simulink model "nms_model_mld"  (R2020a)
settings: Solver=VariableStepAuto  StartTime=0.0  StopTime=10  FixedStep=0.0001  MaxStep=.01  RelTol=1e-4  AbsTol=1e-6
undefined symbols (not defined in the file): animFrameRate, dt_visual, footMass, g, hatLeftHipToCenterDistWidth, hatMass, initialTargetAngle, legMass, LongDelay, LongLoopDelay, LPreStimBFSHinit, LPreStimGASinit, LPreStimGLUinit, LPreStimHABinit, LPreStimHADinit, LPreStimHAMinit, LPreStimHFLinit, LPreStimRFinit, LPreStimSOLinit, LPreStimTAinit, LPreStimVASinit, LTargetAngleInit, LTargetAngleRInit, MidDelay, params, RPreStimBFSHinit, RPreStimGASinit, RPreStimGLUinit, RPreStimHABinit, RPreStimHADinit, RPreStimHAMinit, RPreStimHFLinit, RPreStimRFinit, RPreStimSOLinit, RPreStimTAinit, RPreStimVASinit, RTargetAngleInit, RTargetAngleRInit, shankLength, shankMass, ShortDelay, termination_height, testInterpretedFnc, thetaHATref, thighLength, thighMass, totalMass, X, Y, Z
libraries: NeuroMuscularLibrary x113, nesl_utility x31, sm_lib x25, simulink x3
(part 4 of 5)

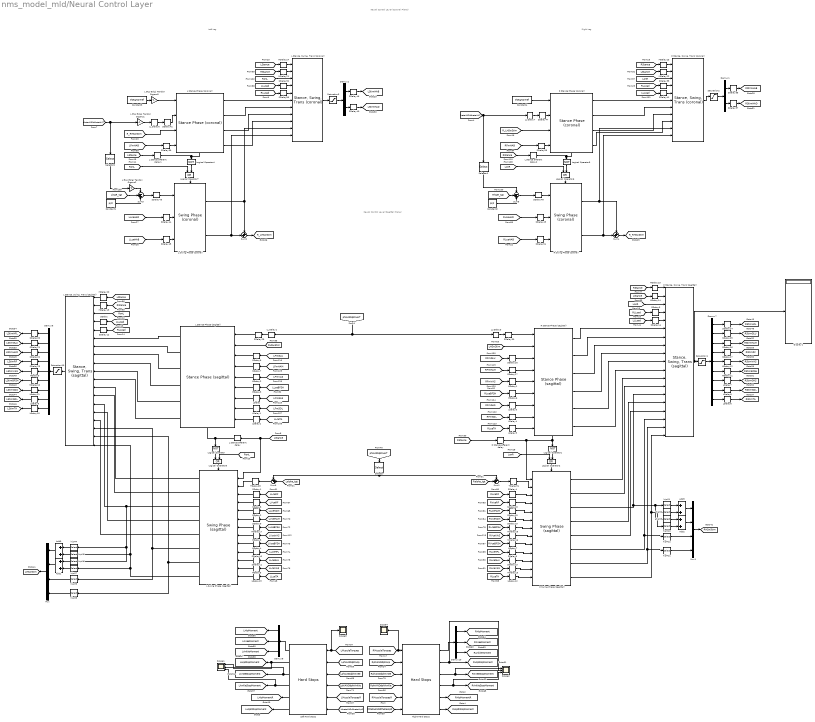
== system nms_model_mld/Neural Control Layer ==
  note: Neural Control Layer
      | (Sagittal Plane)
  note: Neural Control Layer
      | (Coronal Plane)
  note: Right Leg
  note: Left Leg
  Add{1..3,9} (4 alike) : Sum  Inputs=2
  Constant1 : Constant  Value=pi/2
  Constant2 : Constant  Value=pi/2
  Constant3 : Constant  Value=thetaHATref
  Constant4 : Constant  Value=thetaHATref
  Demux1 : Demux  Outputs=2
  Demux10 : Demux  Outputs=3
  Demux2 : Demux  Outputs=2
  Demux6 : Demux  Outputs=9
  Demux7 : Demux  Outputs=9
  Demux8 : Demux  Outputs=3
  Display1 : Display
  L GLU Golgi Tendon Organs1 : Gain  Gain=-1
  L GLU Golgi Tendon Organs2 : Gain  Gain=-1
  L GLU Golgi Tendon Organs3 : Gain  Gain=-1
  L Stance afferent delay : TransportDelay  DelayTime=MidDelay
  L Stance afferent delay1 : TransportDelay  DelayTime=MidDelay
  L Stance afferent delay2 : TransportDelay  DelayTime=MidDelay
  L Stance Phase (coronal) : NeuroMuscularLibrary/Stance Phase (coronal)  PreStimHABst=PreStimHABst  PreStimHADst=PreStimHADst  GainFHABst=GainFHABst  GainPhiHATHABst=GainPhiHATHABst  GainDphiHATHABst=GainDphiHATHABst  GainPhiHATHADst=GainPhiHATHADst  GainDphiHATHADst=GainDphiHATHADst  GainSHABcHABst=GainSHABcHABst  GainSHADcHADst=GainSHADcHADst
  L Stance Phase (sagittal) : NeuroMuscularLibrary/Stance Phase (sagittal)  PreStimHFLst=PreStimHFLst  PreStimGLUst=PreStimGLUst  PreStimHAMst=PreStimHAMst  PreStimRFst=PreStimRFst  PreStimVASst=PreStimVASst  PreStimBFSHst=PreStimBFSHst  PreStimGASst=PreStimGASst  PreStimSOLst=PreStimSOLst  PreStimTAst=PreStimTAst  GainFGLUst=GainFGLUst  GainFVASst=GainFVASst  GainFSOLst=GainFSOLst  GainFHAMst=GainFHAMst  LceOffsetBFSHVASst=LceOffsetBFSHVASst  GainLBFSHVASst=GainLBFSHVASst  LceOffsetBFSHst=LceOffsetBFSHst  GainLBFSHst=GainLBFSHst  GainFGASst=GainFGASst  phiHATref=phiHATref  GainPhiHATHFLst=GainPhiHATHFLst  GainDphiHATHFLst=GainDphiHATHFLst  GainPhiHATGLUst=GainPhiHATGLUst  GainDphiHATGLUst=GainDphiHATGLUst  GainSGLUHAMst=GainSGLUHAMst  GainSGLUcHFLst=GainSGLUcHFLst  GainSHAMcHFLst=GainSHAMcHFLst  GainSHFLcGLUst=GainSHFLcGLUst  GainSRFcGLUst=GainSRFcGLUst  LceOffsetTAst=LceOffsetTAst  GainLTAst=GainLTAst  GainFSOLTAst=GainFSOLTAst
  "L Stance, Swing, Trans (coronal)" : NeuroMuscularLibrary/Stance, Swing, Trans (coronal)  transSupst_C=transSupst_C  transsw_C=transsw_C
  "L Stance, Swing, Trans (sagittal)" : NeuroMuscularLibrary/Stance, Swing, Trans (sagittal)  transSupst=transSupst  transsw=transsw
  L Swing Phase (coronal) : NeuroMuscularLibrary/Swing Phase (coronal)  PreStimHABsw=PreStimHABsw  PreStimHADsw=PreStimHADsw  GainLHABsw=GainLHABsw  GainLHADsw=GainLHADsw
  L Swing Phase (sagittal) : NeuroMuscularLibrary/Swing Phase (sagittal)  PreStimHFLsw=PreStimHFLsw  PreStimGLUsw=PreStimGLUsw  PreStimHAMsw=PreStimHAMsw  PreStimRFsw=PreStimRFsw  PreStimVASsw=PreStimVASsw  PreStimBFSHsw=PreStimBFSHsw  PreStimGASsw=PreStimGASsw  PreStimSOLsw=PreStimSOLsw  PreStimTAsw=PreStimTAsw  GainLTAsw=GainLTAsw  LceOffsetTAsw=LceOffsetTAsw  GainLRFHFLsw=GainLRFHFLsw  GainVRFHFLsw=GainVRFHFLsw  GainLHAMGLUsw=GainLHAMGLUsw  GainVHAMGLUsw=GainVHAMGLUsw  GainVRFBFSHsw=GainVRFBFSHsw  GainVVASRFsw=GainVVASRFsw  GainVBFSHsw=GainVBFSHsw  GainLHAMsw=GainLHAMsw  GainSHAMBFSHsw=GainSHAMBFSHsw  GainSHAMGASsw=GainSHAMGASsw  SHAMthresholdsw=SHAMthresholdsw  GainLHFLsw=GainLHFLsw  GainLGLUsw=GainLGLUsw  LceOffsetVASsw=LceOffsetVASsw  GainLVASsw=GainLVASsw  legLengthClr=legLengthClr  deltaLegAngleThr=deltaLegAngleThr
  LDelay{,1,3..4} (4 alike) : TransportDelay  DelayTime=LongDelay
  LDelay10 : TransportDelay  DelayTime=LongDelay  InitialOutput=LPreStimTAinit
  LDelay11 : TransportDelay  DelayTime=LongDelay  InitialOutput=LPreStimGASinit
  LDelay{2,5,12..13} (4 alike) : TransportDelay  DelayTime=LongDelay  InitialOutput=1
  LDelay6 : TransportDelay  DelayTime=LongDelay  InitialOutput=RPreStimTAinit
  LDelay7 : TransportDelay  DelayTime=LongDelay  InitialOutput=RPreStimGASinit
  LDelay8 : TransportDelay  DelayTime=LongDelay  InitialOutput=RPreStimSOLinit
  LDelay9 : TransportDelay  DelayTime=LongDelay  InitialOutput=LPreStimSOLinit
  LL Delay{2..3,6..7} (4 alike) : TransportDelay  DelayTime=LongLoopDelay/2
  Left Hard Stops : NeuroMuscularLibrary/Hard Stops  SystemSampleTime=-1  Latency=0  AutoFrameSizeCalculation=off
  Logical Operator{,1,4..5} (4 alike) : Logic  Operator=NOT  AllPortsSameDT=off  OutDataTypeStr=boolean
  Logical Operator{2..3,6..7} (4 alike) : Logic  Operator=OR  AllPortsSameDT=off  OutDataTypeStr=boolean
  MDelay{1..2,4,7..8,13..14,16,19..24} (14 alike) : TransportDelay  DelayTime=MidDelay
  MDelay10 : TransportDelay  DelayTime=MidDelay  InitialOutput=LPreStimBFSHinit
  MDelay11 : TransportDelay  DelayTime=MidDelay  InitialOutput=RPreStimBFSHinit
  MDelay12 : TransportDelay  DelayTime=MidDelay  InitialOutput=RPreStimVASinit
  MDelay{3,5..6,15,17..18} (6 alike) : TransportDelay  DelayTime=MidDelay  InitialOutput=1
  MDelay9 : TransportDelay  DelayTime=MidDelay  InitialOutput=LPreStimVASinit
  Mux : Mux
  Mux1 : Mux
  R Stance afferent delay : TransportDelay  DelayTime=MidDelay
  R Stance Phase (coronal) : NeuroMuscularLibrary/Stance Phase (coronal)  PreStimHABst=PreStimHABst  PreStimHADst=PreStimHADst  GainFHABst=GainFHABst  GainPhiHATHABst=GainPhiHATHABst  GainDphiHATHABst=GainDphiHATHABst  GainPhiHATHADst=GainPhiHATHADst  GainDphiHATHADst=GainDphiHATHADst  GainSHABcHABst=GainSHABcHABst  GainSHADcHADst=GainSHADcHADst
  R Stance Phase (sagittal) : NeuroMuscularLibrary/Stance Phase (sagittal)  PreStimHFLst=PreStimHFLst  PreStimGLUst=PreStimGLUst  PreStimHAMst=PreStimHAMst  PreStimRFst=PreStimRFst  PreStimVASst=PreStimVASst  PreStimBFSHst=PreStimBFSHst  PreStimGASst=PreStimGASst  PreStimSOLst=PreStimSOLst  PreStimTAst=PreStimTAst  GainFGLUst=GainFGLUst  GainFVASst=GainFVASst  GainFSOLst=GainFSOLst  GainFHAMst=GainFHAMst  LceOffsetBFSHVASst=LceOffsetBFSHVASst  GainLBFSHVASst=GainLBFSHVASst  LceOffsetBFSHst=LceOffsetBFSHst  GainLBFSHst=GainLBFSHst  GainFGASst=GainFGASst  phiHATref=phiHATref  GainPhiHATHFLst=GainPhiHATHFLst  GainDphiHATHFLst=GainDphiHATHFLst  GainPhiHATGLUst=GainPhiHATGLUst  GainDphiHATGLUst=GainDphiHATGLUst  GainSGLUHAMst=GainSGLUHAMst  GainSGLUcHFLst=GainSGLUcHFLst  GainSHAMcHFLst=GainSHAMcHFLst  GainSHFLcGLUst=GainSHFLcGLUst  GainSRFcGLUst=GainSRFcGLUst  LceOffsetTAst=LceOffsetTAst  GainLTAst=GainLTAst  GainFSOLTAst=GainFSOLTAst
  "R Stance, Swing, Trans (coronal)" : NeuroMuscularLibrary/Stance, Swing, Trans (coronal)  transSupst_C=transSupst_C  transsw_C=transsw_C
  "R Stance, Swing, Trans (sagittal)" : NeuroMuscularLibrary/Stance, Swing, Trans (sagittal)  transSupst=transSupst  transsw=transsw
  R Swing Phase (coronal) : NeuroMuscularLibrary/Swing Phase (coronal)  PreStimHABsw=PreStimHABsw  PreStimHADsw=PreStimHADsw  GainLHABsw=GainLHABsw  GainLHADsw=GainLHADsw
  R Swing Phase (sagittal) : NeuroMuscularLibrary/Swing Phase (sagittal)  PreStimHFLsw=PreStimHFLsw  PreStimGLUsw=PreStimGLUsw  PreStimHAMsw=PreStimHAMsw  PreStimRFsw=PreStimRFsw  PreStimVASsw=PreStimVASsw  PreStimBFSHsw=PreStimBFSHsw  PreStimGASsw=PreStimGASsw  PreStimSOLsw=PreStimSOLsw  PreStimTAsw=PreStimTAsw  GainLTAsw=GainLTAsw  LceOffsetTAsw=LceOffsetTAsw  GainLRFHFLsw=GainLRFHFLsw  GainVRFHFLsw=GainVRFHFLsw  GainLHAMGLUsw=GainLHAMGLUsw  GainVHAMGLUsw=GainVHAMGLUsw  GainVRFBFSHsw=GainVRFBFSHsw  GainVVASRFsw=GainVVASRFsw  GainVBFSHsw=GainVBFSHsw  GainLHAMsw=GainLHAMsw  GainSHAMBFSHsw=GainSHAMBFSHsw  GainSHAMGASsw=GainSHAMGASsw  SHAMthresholdsw=SHAMthresholdsw  GainLHFLsw=GainLHFLsw  GainLGLUsw=GainLGLUsw  LceOffsetVASsw=LceOffsetVASsw  GainLVASsw=GainLVASsw  legLengthClr=legLengthClr  deltaLegAngleThr=deltaLegAngleThr
  Right Hard Stops : NeuroMuscularLibrary/Hard Stops  SystemSampleTime=-1  Latency=0  AutoFrameSizeCalculation=off
  SDelay{,3,6..9,12,14,16..19,29..30,32..33,36,38..39,41..42,47} (22 alike) : TransportDelay  DelayTime=ShortDelay
  SDelay{1..2,4..5,10..11,13,15,34,44..45,49} (12 alike) : TransportDelay  DelayTime=ShortDelay  InitialOutput=1
  SDelay20 : TransportDelay  DelayTime=ShortDelay  InitialOutput=LPreStimHFLinit
  SDelay21 : TransportDelay  DelayTime=ShortDelay  InitialOutput=LPreStimGLUinit
  SDelay22 : TransportDelay  DelayTime=ShortDelay  InitialOutput=LPreStimHAMinit
  SDelay23 : TransportDelay  DelayTime=ShortDelay  InitialOutput=LPreStimRFinit
  SDelay24 : TransportDelay  DelayTime=ShortDelay  InitialOutput=RPreStimHFLinit
  SDelay25 : TransportDelay  DelayTime=ShortDelay  InitialOutput=RPreStimGLUinit
  SDelay26 : TransportDelay  DelayTime=ShortDelay  InitialOutput=RPreStimHAMinit
  SDelay27 : TransportDelay  DelayTime=ShortDelay  InitialOutput=RPreStimRFinit
  SDelay35 : TransportDelay  DelayTime=ShortDelay  InitialOutput=RPreStimHABinit
  SDelay37 : TransportDelay  DelayTime=ShortDelay  InitialOutput=RPreStimHADinit
  SDelay40 : TransportDelay  DelayTime=ShortDelay  InitialOutput=LPreStimHADinit
  SDelay43 : TransportDelay  DelayTime=(ShortDelay + LongLoopDelay/2)  InitialOutput=LTargetAngleRInit
  SDelay46 : TransportDelay  DelayTime=ShortDelay  InitialOutput=LPreStimHABinit
  SDelay48 : TransportDelay  DelayTime=(ShortDelay + LongLoopDelay/2)  InitialOutput=RTargetAngleRInit
  Saturation{1..3,10} (4 alike) : Saturate  UpperLimit=1  LowerLimit=0.01  ZeroCross=off
  Scope1 : Scope  NumInputPorts=3
  Scope2 : Scope  NumInputPorts=3
  Scope3 : Scope
  Scope4 : Scope
  Selector : Selector  InputPortWidth=2  IndexOptions=Index vector (dialog)  Indices=[1]  OutputSizes=1
  Selector1 : Selector  InputPortWidth=2  IndexOptions=Index vector (dialog)  Indices=[1]  OutputSizes=1
  Selector2 : Selector  InputPortWidth=2  IndexOptions=Index vector (dialog)  Indices=[1]  OutputSizes=1
  Sum1 : Sum  Inputs=-+|
  Sum2 : Sum  Inputs=++|
  Sum3 : Sum  Inputs=--+
  Sum4 : Sum  Inputs=++|
  Sum5 : Sum  Inputs=--+
  Sum6 : Sum  Inputs=-+|
  TDelay28 : TransportDelay  DelayTime=(ShortDelay + LongLoopDelay/2)  InitialOutput=LTargetAngleInit
  TDelay31 : TransportDelay  DelayTime=(ShortDelay + LongLoopDelay/2)  InitialOutput=RTargetAngleInit
  hipM{1,4,9,12} (4 alike) : Selector  InputPortWidth=2  IndexOptions=Index vector (dialog)  Indices=1  OutputSizes=1
  hipM10 : Selector  InputPortWidth=3  IndexOptions=Index vector (dialog)  Indices=2  OutputSizes=1
  hipM{2,5,8,11} (4 alike) : Selector  InputPortWidth=3  IndexOptions=Index vector (dialog)  Indices=1  OutputSizes=1
  hipM3 : Selector  InputPortWidth=2  IndexOptions=Index vector (dialog)  Indices=2  OutputSizes=1
  hipM6 : Selector  InputPortWidth=2  IndexOptions=Index vector (dialog)  Indices=2  OutputSizes=1
  hipM7 : Selector  InputPortWidth=3  IndexOptions=Index vector (dialog)  Indices=2  OutputSizes=1
  tag scope: LAnkleMoment=global, LAnkleStopMoment=global, LHSwStim=global, LHipMoment=global, LHipMomentR=global, LHipRStopMoment=global, LHipStopMoment=global, LKneeMoment=global, LKneeStopMoment=global, LStimBFSH=global, LStimGAS=global, LStimGLU=global, LStimHAB=global, LStimHAD=global, LStimHAM=global, LStimHFL=global, LStimRF=global, LStimSOL=global, LStimTA=global, LStimVAS=global, RAnkleMoment=global, RAnkleStopMoment=global, RHSwStim=global, RHipMoment=global, RHipMomentR=global, RHipRStopMoment=global, RHipStopMoment=global, RKneeMoment=global, RKneeStopMoment=global, RStimBFSH=global, RStimGAS=global, RStimGLU=global, RStimHAB=global, RStimHAD=global, RStimHAM=global, RStimHFL=global, RStimRF=global, RStimSOL=global, RStimTA=global, RStimVAS=global, R_LHSwStim=global, R_RHSwStim=global
  wires:
  LDelay11/1 -> [LStimGAS]
  [RLceVAS] -> MDelay15/1
  LDelay10/1 -> [LStimTA]
  L Swing Phase (sagittal)/7 -> "L Stance, Swing, Trans (sagittal)"/18, hipM8/1
  Mux/1 -> [LHSwStim]
  hipM2/1 -> Add3/2
  SDelay11/1 -> L Swing Phase (sagittal)/11
  MDelay16/1 -> R Swing Phase (sagittal)/8
  SDelay24/1 -> [RStimHFL]
  [RLceRF] -> SDelay4/1
  MDelay19/1 -> "L Stance, Swing, Trans (sagittal)"/2
  SDelay10/1 -> L Swing Phase (sagittal)/10
  hipM10/1 -> Add2/2
  R Stance Phase (sagittal)/5 -> "R Stance, Swing, Trans (sagittal)"/10
  hipM4/1 -> Add9/1
  SDelay2/1 -> L Swing Phase (sagittal)/5
  [RLceBFSH] -> MDelay6/1
  [RLceGLU] -> SDelay13/1
  L Swing Phase (sagittal)/1 -> "L Stance, Swing, Trans (sagittal)"/12
  LDelay/1 -> L Stance Phase (sagittal)/7
  L Stance Phase (sagittal)/1 -> "L Stance, Swing, Trans (sagittal)"/6
  SDelay9/1 -> L Swing Phase (sagittal)/6
  L Swing Phase (sagittal)/3 -> "L Stance, Swing, Trans (sagittal)"/14, hipM6/1, hipM4/1
  R Swing Phase (sagittal)/7 -> "R Stance, Swing, Trans (sagittal)"/18, hipM11/1
  R Swing Phase (sagittal)/4 -> "R Stance, Swing, Trans (sagittal)"/15
  Add2/1 -> Mux1/2
  L Swing Phase (sagittal)/5 -> "L Stance, Swing, Trans (sagittal)"/16
  SDelay14/1 -> "R Stance, Swing, Trans (sagittal)"/5
  Demux6/2 -> SDelay21/1
  R Stance Phase (sagittal)/2 -> "R Stance, Swing, Trans (sagittal)"/7
  SDelay12/1 -> "L Stance, Swing, Trans (sagittal)"/5
  MDelay2/1 -> L Stance Phase (sagittal)/5
  Sum1/1 -> TDelay31/1
  Demux7/8 -> LDelay8/1
  hipM6/1 -> Add1/1
  R Stance Phase (sagittal)/3 -> "R Stance, Swing, Trans (sagittal)"/8
  LDelay9/1 -> [LStimSOL]
  Demux6/1 -> SDelay20/1
  L Stance Phase (sagittal)/6 -> "L Stance, Swing, Trans (sagittal)"/11
  SDelay4/1 -> R Swing Phase (sagittal)/3
  [RVceVAS] -> MDelay16/1
  hipM11/1 -> Mux1/4
  MDelay8/1 -> L Swing Phase (sagittal)/8
  Add3/1 -> Mux1/1
  R Swing Phase (sagittal)/6 -> "R Stance, Swing, Trans (sagittal)"/17, hipM12/1
  "R Stance, Swing, Trans (sagittal)"/1 -> Display1/1, Saturation1/1
  [RVceBFSH] -> MDelay7/1
  Add1/1 -> Mux/2
  hipM9/1 -> Mux/3
  L Stance Phase (sagittal)/3 -> "L Stance, Swing, Trans (sagittal)"/8
  LDelay8/1 -> [RStimSOL]
  Logical Operator2/1 -> R Swing Phase (sagittal)/Enable
  hipM5/1 -> Add9/2
  MDelay20/1 -> "L Stance, Swing, Trans (sagittal)"/1
  L Swing Phase (sagittal)/2 -> "L Stance, Swing, Trans (sagittal)"/13
  hipM8/1 -> Mux/4
  L Swing Phase (sagittal)/4 -> "L Stance, Swing, Trans (sagittal)"/15
  L Swing Phase (sagittal)/8 -> "L Stance, Swing, Trans (sagittal)"/19, hipM5/1, hipM7/1
  [LStance] -> MDelay20/1
  R Stance Phase (sagittal)/4 -> "R Stance, Swing, Trans (sagittal)"/9
  LL Delay3/1 -> SDelay30/1
  SDelay30/1 -> R Stance Phase (sagittal)/1
  SDelay22/1 -> [LStimHAM]
  SDelay29/1 -> L Stance Phase (sagittal)/1
  TDelay28/1 -> L Swing Phase (sagittal)/2
  hipM1/1 -> Add3/1
  R Stance Phase (sagittal)/6 -> "R Stance, Swing, Trans (sagittal)"/11
  R Swing Phase (sagittal)/8 -> "R Stance, Swing, Trans (sagittal)"/19, hipM2/1, hipM10/1
  Sum6/1 -> TDelay28/1
  Demux7/1 -> SDelay24/1
  [LLceGLU] -> SDelay11/1
  [RLceHFL] -> SDelay5/1
  L Stance Phase (sagittal)/2 -> "L Stance, Swing, Trans (sagittal)"/7
  R Stance Phase (sagittal)/1 -> "R Stance, Swing, Trans (sagittal)"/6
  [LLceVAS] -> MDelay5/1
  [LHSwStim] -> R Stance Phase (sagittal)/2
  SDelay/1 -> "L Stance, Swing, Trans (sagittal)"/4
  SDelay27/1 -> [RStimRF]
  MDelay11/1 -> [RStimBFSH]
  [RFmSOL] -> LDelay4/1
  MDelay10/1 -> [LStimBFSH]
  Add9/1 -> Mux/1
  [LLceHFL] -> SDelay10/1
  SDelay26/1 -> [RStimHAM]
  SDelay21/1 -> [LStimGLU]
  Demux7/6 -> MDelay11/1
  Demux7/5 -> MDelay12/1
  [LLLoad] -> SDelay14/1
  Saturation1/1 -> Demux7/1
  SDelay5/1 -> R Swing Phase (sagittal)/10
  [LFmSOL] -> LDelay1/1
  hipM12/1 -> Mux1/3
  [LonR] -> "R Stance, Swing, Trans (sagittal)"/3
  MDelay15/1 -> R Swing Phase (sagittal)/12
  [LLLoad] -> SDelay/1
  SDelay25/1 -> [RStimGLU]
  Demux7/3 -> SDelay26/1
  L Stance Phase (sagittal)/4 -> "L Stance, Swing, Trans (sagittal)"/9
  Demux7/4 -> SDelay27/1
  hipM3/1 -> Add2/1
  R Swing Phase (sagittal)/2 -> "R Stance, Swing, Trans (sagittal)"/13
  R Swing Phase (sagittal)/1 -> "R Stance, Swing, Trans (sagittal)"/12
  L Stance Phase (sagittal)/5 -> "L Stance, Swing, Trans (sagittal)"/10
  MDelay9/1 -> [LStimVAS]
  MDelay7/1 -> R Swing Phase (sagittal)/9
  SDelay3/1 -> "R Stance, Swing, Trans (sagittal)"/4
  Demux7/9 -> LDelay6/1
  TDelay31/1 -> R Swing Phase (sagittal)/2
  SDelay19/1 -> R Swing Phase (sagittal)/6
  [RVceHAM] -> SDelay19/1
  SDelay18/1 -> R Swing Phase (sagittal)/4
  SDelay15/1 -> R Swing Phase (sagittal)/5
  [RLceHAM] -> SDelay15/1
  [RLceTA] -> LDelay5/1
  LDelay7/1 -> [RStimGAS]
  LDelay3/1 -> R Stance Phase (sagittal)/7
  [RFmGAS] -> LDelay3/1
  [LLceBFSH] -> MDelay3/1
  [RFmVAS] -> MDelay1/1
  [RLLoad] -> SDelay3/1
  SDelay17/1 -> R Stance Phase (sagittal)/4
  Demux6/7 -> LDelay11/1
  [RStance] -> MDelay19/1
  Saturation10/1 -> Demux6/1
  MDelay4/1 -> L Swing Phase (sagittal)/9
  L Swing Phase (sagittal)/6 -> "L Stance, Swing, Trans (sagittal)"/17, hipM9/1
  Demux6/6 -> MDelay10/1
  Demux6/3 -> SDelay22/1
  LDelay6/1 -> [RStimTA]
  [LVceBFSH] -> MDelay4/1
  SDelay8/1 -> L Swing Phase (sagittal)/4
  Demux6/9 -> LDelay10/1
  [RVceRF] -> SDelay18/1
  Demux6/8 -> LDelay9/1
  Demux6/5 -> MDelay9/1
  MDelay5/1 -> L Swing Phase (sagittal)/12
  SDelay16/1 -> R Stance Phase (sagittal)/3
  SDelay23/1 -> [LStimRF]
  [RLLoad] -> SDelay12/1
  R Swing Phase (sagittal)/3 -> "R Stance, Swing, Trans (sagittal)"/14, hipM3/1, hipM1/1
  [LVceRF] -> SDelay8/1
  SDelay13/1 -> R Swing Phase (sagittal)/11
  Mux1/1 -> [RHSwStim]
  LDelay4/1 -> R Stance Phase (sagittal)/8
  MDelay1/1 -> R Stance Phase (sagittal)/5
  L Stance afferent delay/1 -> L Stance Phase (sagittal)/Enable, Logical Operator/1
  Logical Operator3/1 -> L Swing Phase (sagittal)/Enable
  SDelay20/1 -> [LStimHFL]
  [LLceRF] -> SDelay1/1
  [LVceHAM] -> SDelay9/1
  LDelay2/1 -> L Stance Phase (sagittal)/9
  [LLceTA] -> LDelay2/1
  Demux7/2 -> SDelay25/1
  SDelay1/1 -> L Swing Phase (sagittal)/3
  [RFmHAM] -> SDelay17/1
  Logical Operator/1 -> Logical Operator3/2
  [LLceHAM] -> SDelay2/1
  Demux6/4 -> SDelay23/1
  LDelay1/1 -> L Stance Phase (sagittal)/8
  [LFmGAS] -> LDelay/1
  [RFmGLU] -> SDelay16/1
  MDelay3/1 -> L Stance Phase (sagittal)/6
  SDelay6/1 -> L Stance Phase (sagittal)/3
  [LVceVAS] -> MDelay8/1
  [LFmVAS] -> MDelay2/1
  LL Delay2/1 -> SDelay29/1
  Demux7/7 -> LDelay7/1
  R Swing Phase (sagittal)/5 -> "R Stance, Swing, Trans (sagittal)"/16
  [LFmGLU] -> SDelay6/1
  SDelay7/1 -> L Stance Phase (sagittal)/4
  MDelay6/1 -> R Stance Phase (sagittal)/6
  MDelay12/1 -> [RStimVAS]
  [LFmHAM] -> SDelay7/1
  [RHSwStim] -> L Stance Phase (sagittal)/2
  hipM7/1 -> Add1/2
  Logical Operator1/1 -> Logical Operator2/2
  [RLceTA] -> LDelay12/1
  LDelay12/1 -> R Swing Phase (sagittal)/13
  [LLceTA] -> LDelay13/1
  MDelay17/1 -> L Swing Phase (sagittal)/7
  [LLceBFSH] -> MDelay17/1
  LDelay13/1 -> L Swing Phase (sagittal)/13
  MDelay18/1 -> R Swing Phase (sagittal)/7
  [RLceBFSH] -> MDelay18/1
  LDelay5/1 -> R Stance Phase (sagittal)/9
  R Stance afferent delay/1 -> R Swing Phase (sagittal)/1, R Stance Phase (sagittal)/Enable, Logical Operator1/1
  [RonL] -> "L Stance, Swing, Trans (sagittal)"/3
  [LonR] -> Logical Operator2/1
  [RonL] -> Logical Operator3/1
  [RStance] -> MDelay13/1
  MDelay13/1 -> "R Stance, Swing, Trans (sagittal)"/1
  [LStance] -> MDelay14/1
  MDelay14/1 -> "R Stance, Swing, Trans (sagittal)"/2
  [Ralpha_tgt] -> Sum1/2
  Selector/1 -> Sum6/1, Sum1/1
  [Lalpha_tgt] -> Sum6/2
  [phiANDdphiHAT] -> LL Delay2/1, LL Delay3/1
  [RFmHAB] -> SDelay38/1
  SDelay35/1 -> [RStimHAB]
  [LFmHAB] -> SDelay39/1
  SDelay37/1 -> [RStimHAD]
  [LLceHAD] -> SDelay44/1
  SDelay39/1 -> L Stance Phase (coronal)/4
  L Stance Phase (coronal)/2 -> "L Stance, Swing, Trans (coronal)"/7
  MDelay21/1 -> "L Stance, Swing, Trans (coronal)"/2
  L Swing Phase (coronal)/2 -> "L Stance, Swing, Trans (coronal)"/11, Sum2/2
  [LhipR_tgt] -> Sum3/2
  L GLU Golgi Tendon Organs2/1 -> Sum3/1
  Logical Operator5/1 -> Logical Operator6/2
  [RLceHAD] -> SDelay49/1
  Selector2/1 -> L GLU Golgi Tendon Organs2/1
  Logical Operator4/1 -> Logical Operator7/2
  [LLceHAB] -> SDelay45/1
  Constant4/1 -> R Stance Phase (coronal)/1
  [RonL] -> Logical Operator7/1
  Logical Operator6/1 -> R Swing Phase (coronal)/Enable
  L Swing Phase (coronal)/1 -> "L Stance, Swing, Trans (coronal)"/10, Sum2/1
  L Stance Phase (coronal)/1 -> "L Stance, Swing, Trans (coronal)"/6
  SDelay32/1 -> "L Stance, Swing, Trans (coronal)"/4
  L GLU Golgi Tendon Organs1/1 -> LL Delay6/1
  Sum3/1 -> SDelay43/1
  "L Stance, Swing, Trans (coronal)"/1 -> Saturation3/1
  SDelay43/1 -> L Swing Phase (coronal)/1
  SDelay40/1 -> [LStimHAD]
  MDelay24/1 -> "L Stance, Swing, Trans (coronal)"/1
  Selector1/1 -> Sum5/1
  L Stance afferent delay1/1 -> L Stance Phase (coronal)/Enable, Logical Operator4/1
  SDelay46/1 -> [LStimHAB]
  SDelay45/1 -> L Swing Phase (coronal)/3
  SDelay44/1 -> L Swing Phase (coronal)/2
  [RStance] -> MDelay23/1
  MDelay23/1 -> "R Stance, Swing, Trans (coronal)"/1
  SDelay49/1 -> R Swing Phase (coronal)/2
  [R_LHSwStim] -> R Stance Phase (coronal)/3
  Logical Operator7/1 -> L Swing Phase (coronal)/Enable
  Sum2/1 -> [R_LHSwStim]
  [LStance] -> L Stance afferent delay1/1
  L Stance Phase (coronal)/4 -> "L Stance, Swing, Trans (coronal)"/9
  Demux1/2 -> SDelay37/1
  SDelay42/1 -> L Stance Phase (coronal)/2
  [RonL] -> "L Stance, Swing, Trans (coronal)"/3
  L Stance afferent delay2/1 -> R Stance Phase (coronal)/Enable, Logical Operator5/1
  L Stance Phase (coronal)/3 -> "L Stance, Swing, Trans (coronal)"/8
  SDelay36/1 -> "L Stance, Swing, Trans (coronal)"/5
  Demux2/1 -> SDelay46/1
  [LLLoad] -> SDelay32/1
  [RStance] -> MDelay21/1
  [RLLoad] -> SDelay33/1
  [RStance] -> L Stance afferent delay2/1
  [LStance] -> MDelay24/1
  [LLLoad] -> SDelay41/1
  [LonR] -> Logical Operator6/1
  [RLLoad] -> SDelay36/1
  [R_RHSwStim] -> L Stance Phase (coronal)/3
  L GLU Golgi Tendon Organs3/1 -> L Stance Phase (coronal)/1
  SDelay41/1 -> "R Stance, Swing, Trans (coronal)"/5
  "R Stance, Swing, Trans (coronal)"/1 -> Saturation2/1
  SDelay47/1 -> R Stance Phase (coronal)/2
  Constant2/1 -> Sum5/3
  R Stance Phase (coronal)/2 -> "R Stance, Swing, Trans (coronal)"/7
  SDelay38/1 -> R Stance Phase (coronal)/4
  Saturation2/1 -> Demux1/1
  [LStance] -> MDelay22/1
  SDelay34/1 -> R Swing Phase (coronal)/3
  MDelay22/1 -> "R Stance, Swing, Trans (coronal)"/2
  Constant1/1 -> Sum3/3
  [LonR] -> "R Stance, Swing, Trans (coronal)"/3
  SDelay48/1 -> R Swing Phase (coronal)/1
  [RLceHAB] -> SDelay34/1
  R Stance Phase (coronal)/1 -> "R Stance, Swing, Trans (coronal)"/6
  Saturation3/1 -> Demux2/1
  R Swing Phase (coronal)/1 -> "R Stance, Swing, Trans (coronal)"/10, Sum4/1
  LL Delay7/1 -> SDelay47/1
  R Stance Phase (coronal)/3 -> "R Stance, Swing, Trans (coronal)"/8
  LL Delay6/1 -> SDelay42/1
  R Stance Phase (coronal)/4 -> "R Stance, Swing, Trans (coronal)"/9
  Demux1/1 -> SDelay35/1
  Demux2/2 -> SDelay40/1
  R Swing Phase (coronal)/2 -> "R Stance, Swing, Trans (coronal)"/11, Sum4/2
  SDelay33/1 -> "R Stance, Swing, Trans (coronal)"/4
  Sum4/1 -> [R_RHSwStim]
  [RhipR_tgt] -> Sum5/2
  Constant3/1 -> L GLU Golgi Tendon Organs3/1
  "L Stance, Swing, Trans (sagittal)"/1 -> Saturation10/1
  [RphiANDdphiHip] -> Right Hard Stops/2
  Demux10/2 -> [RKneeMoment]
  [RphiANDdphiAnkle] -> Right Hard Stops/4
  [LMuscleTorques] -> Scope3/1, Left Hard Stops/1
  [LphiANDdphiAnkle] -> Left Hard Stops/4
  [LphiANDdphiKnee] -> Left Hard Stops/3
  [RMuscleTorques] -> Scope4/1, Right Hard Stops/1
  [LphiANDdphiHip] -> Left Hard Stops/2
  Right Hard Stops/1 -> Demux10/1
  Left Hard Stops/1 -> Demux8/1
  Right Hard Stops/3 -> Scope2/2, [RKneeStopMoment]
  Demux10/1 -> [RHipMoment]
  Demux10/3 -> [RAnkleMoment]
  Left Hard Stops/4 -> Scope1/3, [LAnkleStopMoment]
  Right Hard Stops/2 -> Scope2/1, [RHipStopMoment]
  Left Hard Stops/3 -> [LKneeStopMoment], Scope1/2
  Right Hard Stops/4 -> [RAnkleStopMoment], Scope2/3
  Demux8/2 -> [LKneeMoment]
  Left Hard Stops/2 -> Scope1/1, [LHipStopMoment]
  Demux8/1 -> [LHipMoment]
  Demux8/3 -> [LAnkleMoment]
  [RphiANDdphiKnee] -> Right Hard Stops/3
  [LMuscleTorquesR] -> Left Hard Stops/5
  [RMuscleTorquesR] -> Right Hard Stops/5
  Left Hard Stops/5 -> [LHipMomentR]
  Right Hard Stops/5 -> [RHipMomentR]
  [LthetaANDdthetaHipR] -> Left Hard Stops/6
  [RthetaANDdthetaHipR] -> Right Hard Stops/6
  Left Hard Stops/6 -> [LHipRStopMoment]
  Right Hard Stops/6 -> [RHipRStopMoment]
  [phiANDdphiHAT] -> Selector/1
  [thetaANDdthetaHAT] -> LL Delay7/1, Selector1/1
  [thetaANDdthetaHAT] -> L GLU Golgi Tendon Organs1/1, Selector2/1
  [LStance] -> L Swing Phase (sagittal)/1, L Stance afferent delay/1
  [RStance] -> R Stance afferent delay/1
  Sum5/1 -> SDelay48/1

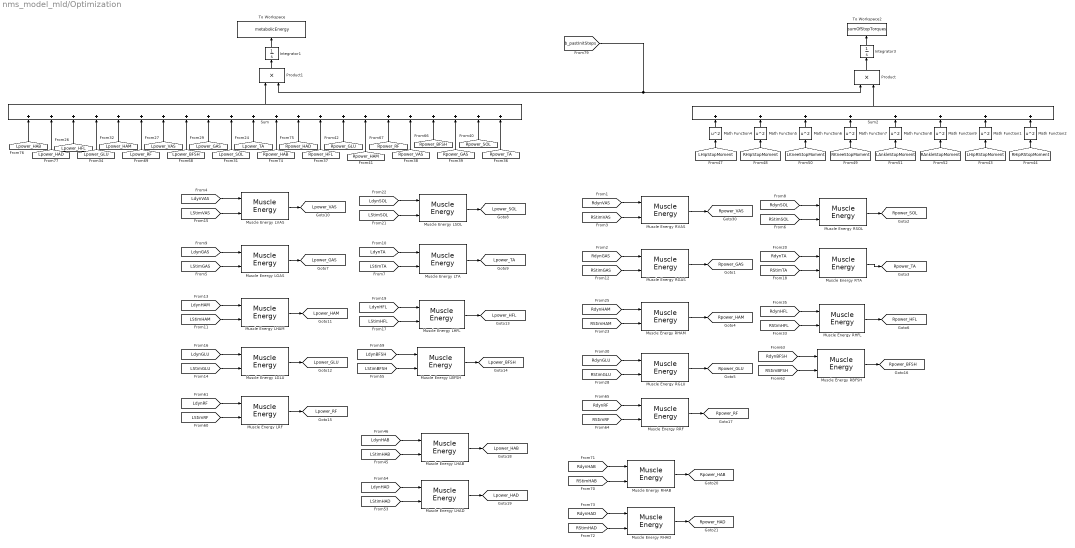
== system nms_model_mld/Optimization ==
  Integrator1 : Integrator
  Integrator3 : Integrator
  Math Function{1..2,4..9} (8 alike) : Math  Operator=square  SignedPower=on  SaturateOnIntegerOverflow=on
  Muscle Energy LBFSH : NeuroMuscularLibrary/Muscle Energy  lopt=loptBFSH  FT=FT_BFSH  Fmax=FmaxBFSH  vmax=vmaxBFSH
  Muscle Energy LGAS : NeuroMuscularLibrary/Muscle Energy  lopt=loptGAS  FT=FT_GAS  Fmax=FmaxGAS  vmax=vmaxGAS
  Muscle Energy LGLU : NeuroMuscularLibrary/Muscle Energy  lopt=loptGLU  FT=FT_GLU  Fmax=FmaxGLU  vmax=vmaxGLU
  Muscle Energy LHAB : NeuroMuscularLibrary/Muscle Energy  lopt=loptHAB  FT=FT_HAB  Fmax=FmaxHAB  vmax=vmaxHAB
  Muscle Energy LHAD : NeuroMuscularLibrary/Muscle Energy  lopt=loptHAD  FT=FT_HAD  Fmax=FmaxHAD  vmax=vmaxHAD
  Muscle Energy LHAM : NeuroMuscularLibrary/Muscle Energy  lopt=loptHAM  FT=FT_HAM  Fmax=FmaxHAM  vmax=vmaxHAM
  Muscle Energy LHFL : NeuroMuscularLibrary/Muscle Energy  lopt=loptHFL  FT=FT_HFL  Fmax=FmaxHFL  vmax=vmaxHFL
  Muscle Energy LRF : NeuroMuscularLibrary/Muscle Energy  lopt=loptRF  FT=FT_RF  Fmax=FmaxRF  vmax=vmaxRF
  Muscle Energy LSOL : NeuroMuscularLibrary/Muscle Energy  lopt=loptSOL  FT=FT_SOL  Fmax=FmaxSOL  vmax=vmaxSOL
  Muscle Energy LTA : NeuroMuscularLibrary/Muscle Energy  lopt=loptTA  FT=FT_TA  Fmax=FmaxTA  vmax=vmaxTA
  Muscle Energy LVAS : NeuroMuscularLibrary/Muscle Energy  lopt=loptVAS  FT=FT_VAS  Fmax=FmaxVAS  vmax=vmaxVAS
  Muscle Energy RBFSH : NeuroMuscularLibrary/Muscle Energy  lopt=loptBFSH  FT=FT_BFSH  Fmax=FmaxBFSH  vmax=vmaxBFSH
  Muscle Energy RGAS : NeuroMuscularLibrary/Muscle Energy  lopt=loptGAS  FT=FT_GAS  Fmax=FmaxGAS  vmax=vmaxGAS
  Muscle Energy RGLU : NeuroMuscularLibrary/Muscle Energy  lopt=loptGLU  FT=FT_GLU  Fmax=FmaxGLU  vmax=vmaxGLU
  Muscle Energy RHAB : NeuroMuscularLibrary/Muscle Energy  lopt=loptHAB  FT=FT_HAB  Fmax=FmaxHAB  vmax=vmaxHAB
  Muscle Energy RHAD : NeuroMuscularLibrary/Muscle Energy  lopt=loptHAD  FT=FT_HAD  Fmax=FmaxHAD  vmax=vmaxHAD
  Muscle Energy RHAM : NeuroMuscularLibrary/Muscle Energy  lopt=loptHAM  FT=FT_HAM  Fmax=FmaxHAM  vmax=vmaxHAM
  Muscle Energy RHFL : NeuroMuscularLibrary/Muscle Energy  lopt=loptHFL  FT=FT_HFL  Fmax=FmaxHFL  vmax=vmaxHFL
  Muscle Energy RRF : NeuroMuscularLibrary/Muscle Energy  lopt=loptRF  FT=FT_RF  Fmax=FmaxRF  vmax=vmaxRF
  Muscle Energy RSOL : NeuroMuscularLibrary/Muscle Energy  lopt=loptSOL  FT=FT_SOL  Fmax=FmaxSOL  vmax=vmaxSOL
  Muscle Energy RTA : NeuroMuscularLibrary/Muscle Energy  lopt=loptTA  FT=FT_TA  Fmax=FmaxTA  vmax=vmaxTA
  Muscle Energy RVAS : NeuroMuscularLibrary/Muscle Energy  lopt=loptVAS  FT=FT_VAS  Fmax=FmaxVAS  vmax=vmaxVAS
  Product : Product
  Product1 : Product
  Sum : Sum  Inputs=++++++++++++++++++++++
  Sum2 : Sum  Inputs=++++++++
  To Workspace : ToWorkspace  VariableName=metabolicEnergy  SampleTime=-1
      settings: MaxDataPoints=1
  To Workspace2 : ToWorkspace  VariableName=sumOfStopTorques  SampleTime=-1
      settings: MaxDataPoints=1
  tag scope: Lpower_BFSH=global, Lpower_GAS=global, Lpower_GLU=global, Lpower_HAB=global, Lpower_HAD=global, Lpower_HAM=global, Lpower_HFL=global, Lpower_RF=global, Lpower_SOL=global, Lpower_TA=global, Lpower_VAS=global, Rpower_BFSH=global, Rpower_GAS=global, Rpower_GLU=global, Rpower_HAB=global, Rpower_HAD=global, Rpower_HAM=global, Rpower_HFL=global, Rpower_RF=global, Rpower_SOL=global, Rpower_TA=global, Rpower_VAS=global
  wires:
  [RdynSOL] -> Muscle Energy RSOL/1
  [RStimSOL] -> Muscle Energy RSOL/2
  [RStimVAS] -> Muscle Energy RVAS/2
  [RStimGAS] -> Muscle Energy RGAS/2
  Muscle Energy RVAS/1 -> [Rpower_VAS]
  Muscle Energy RGAS/1 -> [Rpower_GAS]
  Muscle Energy RSOL/1 -> [Rpower_SOL]
  Muscle Energy RTA/1 -> [Rpower_TA]
  [RdynTA] -> Muscle Energy RTA/1
  [RStimTA] -> Muscle Energy RTA/2
  [RdynHAM] -> Muscle Energy RHAM/1
  [RStimHAM] -> Muscle Energy RHAM/2
  [RdynGLU] -> Muscle Energy RGLU/1
  [RStimGLU] -> Muscle Energy RGLU/2
  [RdynHFL] -> Muscle Energy RHFL/1
  [RStimHFL] -> Muscle Energy RHFL/2
  Muscle Energy RHAM/1 -> [Rpower_HAM]
  Muscle Energy RGLU/1 -> [Rpower_GLU]
  Muscle Energy RHFL/1 -> [Rpower_HFL]
  [Lpower_HAB] -> Sum/1
  [Lpower_VAS] -> Sum/7
  [Lpower_RF] -> Sum/6
  [Lpower_HAM] -> Sum/5
  [Lpower_GLU] -> Sum/4
  [Lpower_HFL] -> Sum/3
  [Lpower_HAD] -> Sum/2
  [RdynGAS] -> Muscle Energy RGAS/1
  [RdynVAS] -> Muscle Energy RVAS/1
  [LdynSOL] -> Muscle Energy LSOL/1
  [LStimSOL] -> Muscle Energy LSOL/2
  [LStimVAS] -> Muscle Energy LVAS/2
  [LStimGAS] -> Muscle Energy LGAS/2
  Muscle Energy LVAS/1 -> [Lpower_VAS]
  Muscle Energy LGAS/1 -> [Lpower_GAS]
  Muscle Energy LSOL/1 -> [Lpower_SOL]
  Muscle Energy LTA/1 -> [Lpower_TA]
  [LdynTA] -> Muscle Energy LTA/1
  [LStimTA] -> Muscle Energy LTA/2
  [LdynHAM] -> Muscle Energy LHAM/1
  [LStimHAM] -> Muscle Energy LHAM/2
  [LdynGLU] -> Muscle Energy LGLU/1
  [LStimGLU] -> Muscle Energy LGLU/2
  [LdynHFL] -> Muscle Energy LHFL/1
  [LStimHFL] -> Muscle Energy LHFL/2
  Muscle Energy LHAM/1 -> [Lpower_HAM]
  Muscle Energy LGLU/1 -> [Lpower_GLU]
  Muscle Energy LHFL/1 -> [Lpower_HFL]
  [LdynGAS] -> Muscle Energy LGAS/1
  [LdynVAS] -> Muscle Energy LVAS/1
  [Lpower_SOL] -> Sum/10
  [Rpower_HAM] -> Sum/16
  [Rpower_GLU] -> Sum/15
  [Rpower_HFL] -> Sum/14
  [Rpower_HAD] -> Sum/13
  [Rpower_HAB] -> Sum/12
  [Lpower_TA] -> Sum/11
  Integrator1/1 -> To Workspace/1
  Sum/1 -> Product1/1
  Integrator3/1 -> To Workspace2/1
  Math Function4/1 -> Sum2/1
  [LHipStopMoment] -> Math Function4/1
  Math Function5/1 -> Sum2/2
  [RHipStopMoment] -> Math Function5/1
  Math Function6/1 -> Sum2/3
  Math Function7/1 -> Sum2/4
  [LKneeStopMoment] -> Math Function6/1
  [RKneeStopMoment] -> Math Function7/1
  [LAnkleStopMoment] -> Math Function8/1
  Math Function8/1 -> Sum2/5
  [RAnkleStopMoment] -> Math Function9/1
  Math Function9/1 -> Sum2/6
  Product/1 -> Integrator3/1
  Sum2/1 -> Product/2
  Product1/1 -> Integrator1/1
  Muscle Energy LBFSH/1 -> [Lpower_BFSH]
  [LStimBFSH] -> Muscle Energy LBFSH/2
  [LdynBFSH] -> Muscle Energy LBFSH/1
  [LdynRF] -> Muscle Energy LRF/1
  [LStimRF] -> Muscle Energy LRF/2
  Muscle Energy LRF/1 -> [Lpower_RF]
  Muscle Energy RRF/1 -> [Rpower_RF]
  [RdynRF] -> Muscle Energy RRF/1
  Muscle Energy RBFSH/1 -> [Rpower_BFSH]
  [RStimRF] -> Muscle Energy RRF/2
  [RStimBFSH] -> Muscle Energy RBFSH/2
  [RdynBFSH] -> Muscle Energy RBFSH/1
  [Lpower_BFSH] -> Sum/8
  [Lpower_GAS] -> Sum/9
  [Rpower_VAS] -> Sum/18
  [Rpower_RF] -> Sum/17
  Math Function1/1 -> Sum2/7
  [LHipRStopMoment] -> Math Function1/1
  [RHipRStopMoment] -> Math Function2/1
  Muscle Energy LHAB/1 -> [Lpower_HAB]
  [LStimHAB] -> Muscle Energy LHAB/2
  [LdynHAB] -> Muscle Energy LHAB/1
  [LdynHAD] -> Muscle Energy LHAD/1
  [LStimHAD] -> Muscle Energy LHAD/2
  Muscle Energy LHAD/1 -> [Lpower_HAD]
  Muscle Energy RHAD/1 -> [Rpower_HAD]
  [RStimHAD] -> Muscle Energy RHAD/2
  [RdynHAD] -> Muscle Energy RHAD/1
  [RdynHAB] -> Muscle Energy RHAB/1
  [RStimHAB] -> Muscle Energy RHAB/2
  Muscle Energy RHAB/1 -> [Rpower_HAB]
  [Rpower_TA] -> Sum/22
  [Rpower_SOL] -> Sum/21
  [Rpower_GAS] -> Sum/20
  [Rpower_BFSH] -> Sum/19
  Math Function2/1 -> Sum2/8
  [b_pastInitSteps] -> Product/1, Product1/2

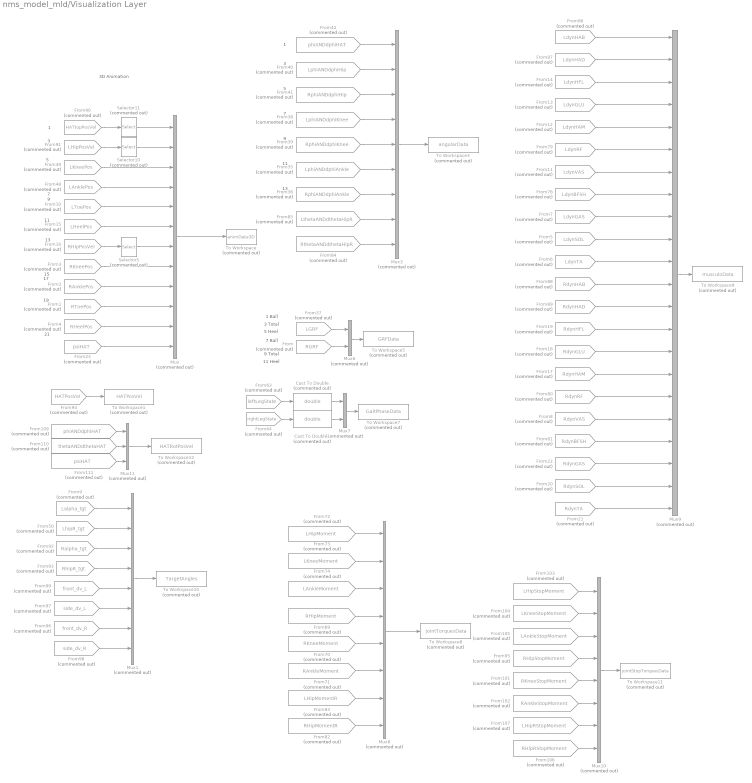
== system nms_model_mld/Visualization Layer ==
  note: 21
  note: 19
  note: 17
  note: 15
  note: 13
  note: 11
  note: 9
  note: 7
  note: 5
  note: 3
  note: 1
  note: 3D Animation
  note: 1
  note: 13
  note: 3
  note: 5
  note: 7
  note: 9
  note: 11
  note: 9 Total
  note: 1 Ball
  note: 5 Heel
  note: 11 Heel
  note: 3 Total
  note: 7 Ball
  Cast To Double : DataTypeConversion  Commented=on  OutDataTypeStr=double
  Cast To Double1 : DataTypeConversion  Commented=on  OutDataTypeStr=double
  From : From  Commented=on  GotoTag=RGRF  TagVisibility=global
  From1 : From  Commented=on  GotoTag=RToePos  TagVisibility=global
      settings: CloseFcn=tagdialog Close
  From10 : From  Commented=on  GotoTag=LToePos  TagVisibility=global
      settings: CloseFcn=tagdialog Close
  From101 : From  Commented=on  GotoTag=RKneeStopMoment  TagVisibility=global
  From102 : From  Commented=on  GotoTag=RAnkleStopMoment  TagVisibility=global
  From103 : From  Commented=on  GotoTag=LHipStopMoment  TagVisibility=global
  From104 : From  Commented=on  GotoTag=LKneeStopMoment  TagVisibility=global
  From105 : From  Commented=on  GotoTag=LAnkleStopMoment  TagVisibility=global
  From106 : From  Commented=on  GotoTag=RHipRStopMoment  TagVisibility=global
  From107 : From  Commented=on  GotoTag=LHipRStopMoment  TagVisibility=global
  From109 : From  Commented=on  GotoTag=phiANDdphiHAT  TagVisibility=global
  From11 : From  Commented=on  GotoTag=LdynVAS  TagVisibility=global
  From110 : From  Commented=on  GotoTag=thetaANDdthetaHAT  TagVisibility=global
  From111 : From  Commented=on  GotoTag=psiHAT  TagVisibility=global
  From12 : From  Commented=on  GotoTag=LdynHAM  TagVisibility=global
  From13 : From  Commented=on  GotoTag=LdynGLU  TagVisibility=global
  From14 : From  Commented=on  GotoTag=LdynHFL  TagVisibility=global
  From15 : From  Commented=on  GotoTag=LHeelPos  TagVisibility=global
      settings: CloseFcn=tagdialog Close
  From16 : From  Commented=on  GotoTag=RHipPosVel  TagVisibility=global
  From17 : From  Commented=on  GotoTag=RdynHAM  TagVisibility=global
  From18 : From  Commented=on  GotoTag=RdynGLU  TagVisibility=global
  From19 : From  Commented=on  GotoTag=RdynHFL  TagVisibility=global
  From2 : From  Commented=on  GotoTag=RAnklePos  TagVisibility=global
      settings: CloseFcn=tagdialog Close
  From20 : From  Commented=on  GotoTag=RdynSOL  TagVisibility=global
  From21 : From  Commented=on  GotoTag=RdynTA  TagVisibility=global
  From22 : From  Commented=on  GotoTag=RdynGAS  TagVisibility=global
  From23 : From  Commented=on  GotoTag=psiHAT  TagVisibility=global
  From3 : From  Commented=on  GotoTag=RKneePos  TagVisibility=global
      settings: CloseFcn=tagdialog Close
  From35 : From  Commented=on  GotoTag=LphiANDdphiAnkle  TagVisibility=global
  From36 : From  Commented=on  GotoTag=RphiANDdphiAnkle  TagVisibility=global
  From37 : From  Commented=on  GotoTag=LGRF  TagVisibility=global
  From38 : From  Commented=on  GotoTag=LphiANDdphiKnee  TagVisibility=global
  From39 : From  Commented=on  GotoTag=RphiANDdphiKnee  TagVisibility=global
  From4 : From  Commented=on  GotoTag=RHeelPos  TagVisibility=global
      settings: CloseFcn=tagdialog Close
  From40 : From  Commented=on  GotoTag=LphiANDdphiHip  TagVisibility=global
  From41 : From  Commented=on  GotoTag=RphiANDdphiHip  TagVisibility=global
  From42 : From  Commented=on  GotoTag=phiANDdphiHAT  TagVisibility=global
  From48 : From  Commented=on  GotoTag=LAnklePos  TagVisibility=global
      settings: CloseFcn=tagdialog Close
  From49 : From  Commented=on  GotoTag=LKneePos  TagVisibility=global
      settings: CloseFcn=tagdialog Close
  From5 : From  Commented=on  GotoTag=LdynSOL  TagVisibility=global
  From50 : From  Commented=on  GotoTag=LhipR_tgt  TagVisibility=global
  From6 : From  Commented=on  GotoTag=LdynTA  TagVisibility=global
  From63 : From  Commented=on  GotoTag=leftLegState  TagVisibility=global
  From64 : From  Commented=on  GotoTag=rightLegState  TagVisibility=global
  From69 : From  Commented=on  GotoTag=RHipMoment  TagVisibility=global
  From7 : From  Commented=on  GotoTag=LdynGAS  TagVisibility=global
  From70 : From  Commented=on  GotoTag=RKneeMoment  TagVisibility=global
  From71 : From  Commented=on  GotoTag=RAnkleMoment  TagVisibility=global
  From72 : From  Commented=on  GotoTag=LHipMoment  TagVisibility=global
  From73 : From  Commented=on  GotoTag=LKneeMoment  TagVisibility=global
  From74 : From  Commented=on  GotoTag=LAnkleMoment  TagVisibility=global
  From78 : From  Commented=on  GotoTag=LdynBFSH  TagVisibility=global
  From79 : From  Commented=on  GotoTag=LdynRF  TagVisibility=global
  From8 : From  Commented=on  GotoTag=RdynVAS  TagVisibility=global
  From80 : From  Commented=on  GotoTag=RdynRF  TagVisibility=global
  From81 : From  Commented=on  GotoTag=RdynBFSH  TagVisibility=global
  From82 : From  Commented=on  GotoTag=RHipMomentR  TagVisibility=global
  From83 : From  Commented=on  GotoTag=LHipMomentR  TagVisibility=global
  From84 : From  Commented=on  GotoTag=RthetaANDdthetaHipR  TagVisibility=global
  From85 : From  Commented=on  GotoTag=LthetaANDdthetaHipR  TagVisibility=global
  From86 : From  Commented=on  GotoTag=LdynHAB  TagVisibility=global
  From87 : From  Commented=on  GotoTag=LdynHAD  TagVisibility=global
  From88 : From  Commented=on  GotoTag=RdynHAB  TagVisibility=global
  From89 : From  Commented=on  GotoTag=RdynHAD  TagVisibility=global
  From9 : From  Commented=on  GotoTag=Lalpha_tgt  TagVisibility=global
  From90 : From  Commented=on  GotoTag=HATtopPosVel  TagVisibility=global
  From91 : From  Commented=on  GotoTag=LHipPosVel  TagVisibility=global
  From92 : From  Commented=on  GotoTag=Ralpha_tgt  TagVisibility=global
  From93 : From  Commented=on  GotoTag=RhipR_tgt  TagVisibility=global
  From94 : From  Commented=on  GotoTag=HATPosVel  TagVisibility=global
  From95 : From  Commented=on  GotoTag=RHipStopMoment  TagVisibility=global
  From96 : From  Commented=on  GotoTag=front_dv_R  TagVisibility=global
      settings: CloseFcn=tagdialog Close
  From97 : From  Commented=on  GotoTag=side_dv_L  TagVisibility=global
      settings: CloseFcn=tagdialog Close
  From98 : From  Commented=on  GotoTag=side_dv_R  TagVisibility=global
      settings: CloseFcn=tagdialog Close
  From99 : From  Commented=on  GotoTag=front_dv_L  TagVisibility=global
      settings: CloseFcn=tagdialog Close
  Mux : Mux  Commented=on  Inputs=12
  Mux1 : Mux  Commented=on  Inputs=8
  Mux10 : Mux  Commented=on  Inputs=8
  Mux11 : Mux  Commented=on  Inputs=3
  Mux3 : Mux  Commented=on  Inputs=9
  Mux6 : Mux  Commented=on  Inputs=2
  Mux7 : Mux  Commented=on  Inputs=2
  Mux8 : Mux  Commented=on  Inputs=8
  Mux9 : Mux  Commented=on  Inputs=22
  Selector10 : Selector  Commented=on  InputPortWidth=6  IndexOptions=Index vector (dialog)  Indices=[1 2 3]  OutputSizes=1
  Selector11 : Selector  Commented=on  InputPortWidth=6  IndexOptions=Index vector (dialog)  Indices=[1 2 3]  OutputSizes=1
  Selector5 : Selector  Commented=on  InputPortWidth=6  IndexOptions=Index vector (dialog)  Indices=[1 2 3]  OutputSizes=1
  To Workspace : ToWorkspace  Commented=on  VariableName=animData3D  SaveFormat=Structure With Time  SampleTime=1/animFrameRate
  To Workspace1 : ToWorkspace  Commented=on  VariableName=HATPosVel  SaveFormat=Structure With Time  SampleTime=dt_visual
  To Workspace10 : ToWorkspace  Commented=on  VariableName=TargetAngles  SaveFormat=Structure With Time  SampleTime=dt_visual
  To Workspace11 : ToWorkspace  Commented=on  VariableName=jointStopTorquesData  SaveFormat=Structure With Time  SampleTime=dt_visual
  To Workspace12 : ToWorkspace  Commented=on  VariableName=HATRotPosVel  SaveFormat=Structure With Time  SampleTime=dt_visual
  To Workspace3 : ToWorkspace  Commented=on  VariableName=angularData  SaveFormat=Structure With Time  SampleTime=dt_visual
  To Workspace5 : ToWorkspace  Commented=on  VariableName=GRFData  SaveFormat=Structure With Time  SampleTime=dt_visual
  To Workspace7 : ToWorkspace  Commented=on  VariableName=GaitPhaseData  SaveFormat=Structure With Time  SampleTime=dt_visual
  To Workspace8 : ToWorkspace  Commented=on  VariableName=jointTorquesData  SaveFormat=Structure With Time  SampleTime=dt_visual
  To Workspace9 : ToWorkspace  Commented=on  VariableName=musculoData  SaveFormat=Structure With Time  SampleTime=dt_visual
  wires:
  From16/1 -> Selector5/1
  From90/1 -> Selector11/1
  From91/1 -> Selector10/1
  Selector11/1 -> Mux/1
  From2/1 -> Mux/9
  From3/1 -> Mux/8
  Selector5/1 -> Mux/7
  From15/1 -> Mux/6
  From10/1 -> Mux/5
  From48/1 -> Mux/4
  From49/1 -> Mux/3
  Selector10/1 -> Mux/2
  Mux/1 -> To Workspace/1
  From4/1 -> Mux/11
  From1/1 -> Mux/10
  From36/1 -> Mux3/7
  Mux6/1 -> To Workspace5/1
  From/1 -> Mux6/2
  From42/1 -> Mux3/1
  Mux3/1 -> To Workspace3/1
  From35/1 -> Mux3/6
  From38/1 -> Mux3/4
  From37/1 -> Mux6/1
  From40/1 -> Mux3/2
  From39/1 -> Mux3/5
  From41/1 -> Mux3/3
  From64/1 -> Cast To Double1/1
  Mux7/1 -> To Workspace7/1
  From63/1 -> Cast To Double/1
  Mux8/1 -> To Workspace8/1
  From72/1 -> Mux8/1
  From73/1 -> Mux8/2
  From74/1 -> Mux8/3
  From69/1 -> Mux8/4
  From70/1 -> Mux8/5
  From71/1 -> Mux8/6
  Mux9/1 -> To Workspace9/1
  From17/1 -> Mux9/16
  From14/1 -> Mux9/3
  From18/1 -> Mux9/15
  From8/1 -> Mux9/18
  From78/1 -> Mux9/8
  From22/1 -> Mux9/20
  From81/1 -> Mux9/19
  From11/1 -> Mux9/7
  From7/1 -> Mux9/9
  From5/1 -> Mux9/10
  From79/1 -> Mux9/6
  From12/1 -> Mux9/5
  From13/1 -> Mux9/4
  From6/1 -> Mux9/11
  From80/1 -> Mux9/17
  From19/1 -> Mux9/14
  From20/1 -> Mux9/21
  From21/1 -> Mux9/22
  From83/1 -> Mux8/7
  From82/1 -> Mux8/8
  From85/1 -> Mux3/8
  From84/1 -> Mux3/9
  From88/1 -> Mux9/12
  From89/1 -> Mux9/13
  From86/1 -> Mux9/1
  From87/1 -> Mux9/2
  From94/1 -> To Workspace1/1
  From99/1 -> Mux1/5
  From92/1 -> Mux1/3
  From93/1 -> Mux1/4
  Mux1/1 -> To Workspace10/1
  From96/1 -> Mux1/7
  From50/1 -> Mux1/2
  From98/1 -> Mux1/8
  From97/1 -> Mux1/6
  From9/1 -> Mux1/1
  From102/1 -> Mux10/6
  From95/1 -> Mux10/4
  From104/1 -> Mux10/2
  Mux10/1 -> To Workspace11/1
  From103/1 -> Mux10/1
  From101/1 -> Mux10/5
  From105/1 -> Mux10/3
  From107/1 -> Mux10/7
  From106/1 -> Mux10/8
  Mux11/1 -> To Workspace12/1
  From110/1 -> Mux11/2
  From111/1 -> Mux11/3
  From109/1 -> Mux11/1
  From23/1 -> Mux/12
  Cast To Double/1 -> Mux7/1
  Cast To Double1/1 -> Mux7/2

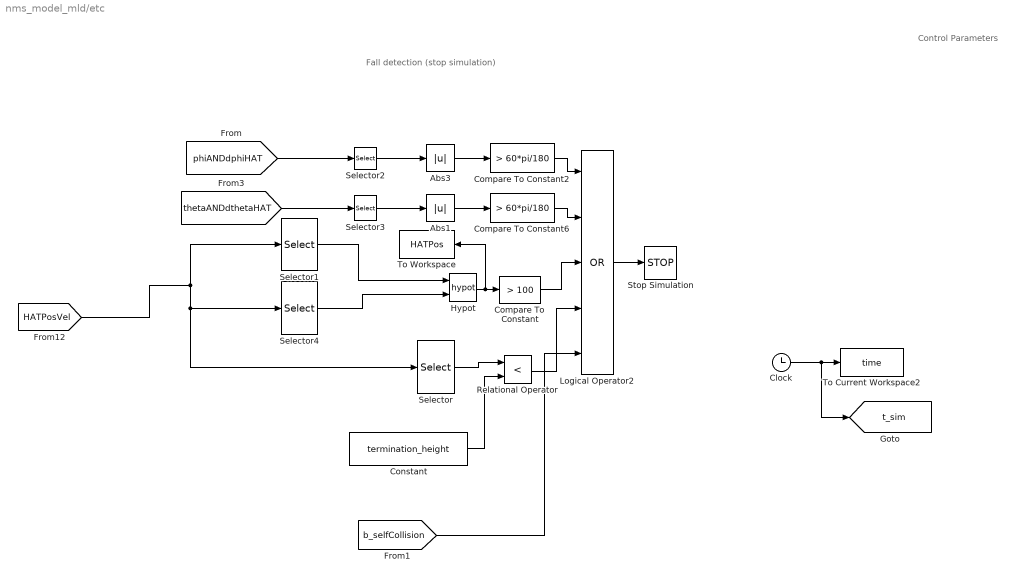
== system nms_model_mld/etc ==
  note: Fall detection
      | (stop simulation)
  note: Control Parameters
  Abs1 : Abs
  Abs3 : Abs
  Clock : Clock
  Compare To Constant : simulink/Logic and Bit Operations/Compare To Constant  relop=>  const=100  OutDataTypeStr=boolean
  Compare To Constant2 : simulink/Logic and Bit Operations/Compare To Constant  relop=>  const=60*pi/180  OutDataTypeStr=boolean
  Compare To Constant6 : simulink/Logic and Bit Operations/Compare To Constant  relop=>  const=60*pi/180  OutDataTypeStr=boolean
  Constant : Constant  Value=termination_height
  Hypot : Math  Operator=hypot  SaturateOnIntegerOverflow=on
  Logical Operator2 : Logic  Operator=OR  Inputs=5  AllPortsSameDT=off  OutDataTypeStr=boolean
  Relational Operator : RelationalOperator  Operator=<  OutDataTypeStr=boolean  RndMeth=Nearest
  Selector : Selector  InputPortWidth=6  IndexOptions=Index vector (dialog)  Indices=[3]  OutputSizes=1
  Selector1 : Selector  InputPortWidth=6  IndexOptions=Index vector (dialog)  Indices=[1]  OutputSizes=1
  Selector2 : Selector  InputPortWidth=2  IndexOptions=Index vector (dialog)  Indices=[1]  OutputSizes=1
  Selector3 : Selector  InputPortWidth=2  IndexOptions=Index vector (dialog)  Indices=[1]  OutputSizes=1
  Selector4 : Selector  InputPortWidth=6  IndexOptions=Index vector (dialog)  Indices=[2]  OutputSizes=1
  Stop Simulation : Stop
  To Current Workspace2 : ToWorkspace  VariableName=time  SampleTime=-1
      settings: MaxDataPoints=1
  To Workspace : ToWorkspace  VariableName=HATPos  SampleTime=-1
      settings: MaxDataPoints=1
  tag scope: t_sim=global
  wires:
  Selector2/1 -> Abs3/1
  Abs3/1 -> Compare To Constant2/1
  Compare To Constant2/1 -> Logical Operator2/1
  Logical Operator2/1 -> Stop Simulation/1
  Selector3/1 -> Abs1/1
  Abs1/1 -> Compare To Constant6/1
  Compare To Constant6/1 -> Logical Operator2/2
  Compare To Constant/1 -> Logical Operator2/3
  Selector/1 -> Relational Operator/1
  Selector1/1 -> Hypot/1
  Constant/1 -> Relational Operator/2
  Relational Operator/1 -> Logical Operator2/4
  [HATPosVel] -> Selector1/1, Selector/1, Selector4/1
  Clock/1 -> [t_sim], To Current Workspace2/1
  [phiANDdphiHAT] -> Selector2/1
  [thetaANDdthetaHAT] -> Selector3/1
  Selector4/1 -> Hypot/2
  Hypot/1 -> To Workspace/1, Compare To Constant/1
  [b_selfCollision] -> Logical Operator2/5

== system nms_model_mld/Body Mechanics Layer/CMG Thigh ==
  Constant : Constant  Value=0
  External Force and Torque : sm_lib/Forces and Torques/External Force and Torque  ForceResolutionFrame=AttachedFrame  EnableForceX=off  EnableForceY=off  EnableForceZ=off  EnableForce=off  TorqueResolutionFrame=AttachedFrame  EnableTorqueX=on  EnableTorqueY=off  EnableTorqueZ=off  EnableTorque=off
  Simulink-PS Converter8 : nesl_utility/Simulink-PS Converter  PhysicalDomain=network_engine_domain  SubClassName=ps_input  LeftPortType=input  RightPortType=output  PseudoPeriodic=off  Frequencies=[]  NoiseDistribution=none  NoiseParameters=[]  Unit=N*m  AffineConversion=off  FilteringAndDerivatives=provide  SimscapeFilterOrder=1  InputFilterTimeConstant=0.001  UdotUserProvided=0
  External Force and Torque1 : PMIOPort  Side=Right
  wires:
  Constant/1 -> Simulink-PS Converter8/1
  connections:
  Simulink-PS Converter8/RConn1 -- External Force and Torque/LConn1
  External Force and Torque/RConn1 -- External Force and Torque1/RConn1

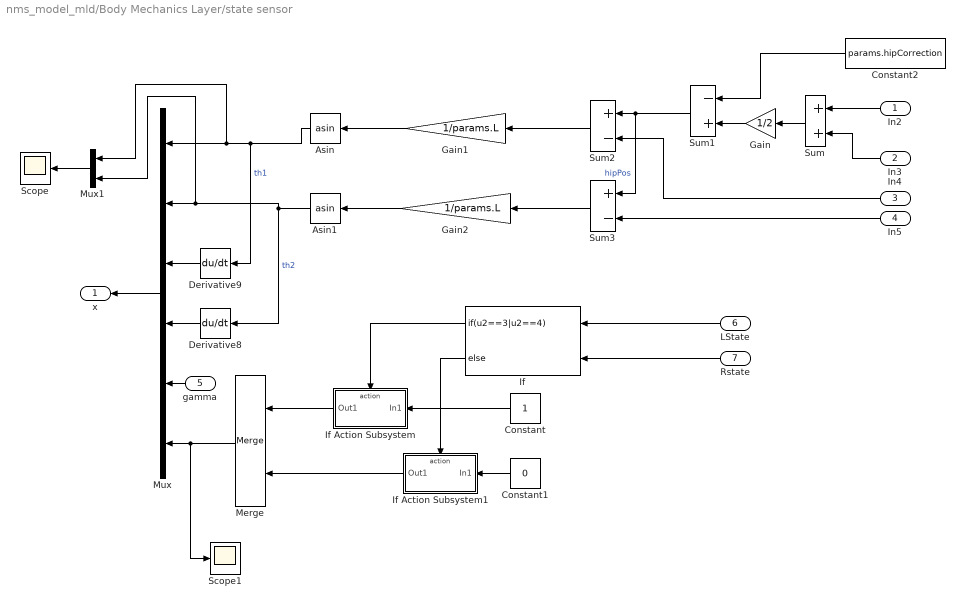
== system nms_model_mld/Body Mechanics Layer/state sensor ==
  In2 : Inport
  In3 : Inport  Port=2
  In4 : Inport  Port=3
  In5 : Inport  Port=4
  gamma : Inport  Port=5
  LState : Inport  Port=6
  Rstate : Inport  Port=7
  Asin : Trigonometry  Operator=asin
  Asin1 : Trigonometry  Operator=asin
  Constant : Constant
  Constant1 : Constant  Value=0
  Constant2 : Constant  Value=params.hipCorrection
  Derivative8 : Derivative
  Derivative9 : Derivative
  Gain : Gain  Gain=1/2
  Gain1 : Gain  Gain=1/params.L
  Gain2 : Gain  Gain=1/params.L
  If : If  NumInputs=2  IfExpression=u2==3|u2==4
  If Action Subsystem : Subsystem  TreatAsAtomicUnit=on
  If Action Subsystem1 : Subsystem  TreatAsAtomicUnit=on
  Merge : Merge
  Mux : Mux  Inputs=6
  Mux1 : Mux  Inputs=2
  Scope : Scope
  Scope1 : Scope
  Sum : Sum
  Sum1 : Sum  Inputs=-+
  Sum2 : Sum  Inputs=+-
  Sum3 : Sum  Inputs=+-
  x : Outport  PortDimensions=6
  wires:
  Gain2/1 -> Asin1/1
  Sum3/1 -> Gain2/1
  Gain/1 -> Sum1/2
  Gain1/1 -> Asin/1
  Sum1/1 -> Sum3/1, Sum2/1  "hipPos"
  Asin/1 -> Derivative9/1, Mux1/1, Mux/1  "th1"
  Asin1/1 -> Derivative8/1, Mux1/2, Mux/2  "th2"
  Sum/1 -> Gain/1
  In2/1 -> Sum/1
  Sum2/1 -> Gain1/1
  In4/1 -> Sum2/2
  In5/1 -> Sum3/2
  In3/1 -> Sum/2
  Constant2/1 -> Sum1/1
  Derivative9/1 -> Mux/3
  Derivative8/1 -> Mux/4
  Mux/1 -> x/1
  LState/1 -> If/1
  Rstate/1 -> If/2
  Constant1/1 -> If Action Subsystem1/1(In1)
  Constant/1 -> If Action Subsystem/1(In1)
  If Action Subsystem1/1(Out1) -> Merge/2
  If Action Subsystem/1(Out1) -> Merge/1
  If/1 -> If Action Subsystem/Action
  If/2 -> If Action Subsystem1/Action
  Merge/1 -> Scope1/1, Mux/6
  gamma/1 -> Mux/5
  Mux1/1 -> Scope/1

== system nms_model_mld/Control Moment Gyroscope/If Action Subsystem ==
  In1 : Inport
  Action Port : ActionPort  ActionPortLabel=if(u1<3 &(u2==0|u2>2))
  Out1 : Outport
  wires:
  In1/1 -> Out1/1

== system nms_model_mld/Control Moment Gyroscope/If Action Subsystem1 ==
  In1 : Inport
  Action Port : ActionPort  ActionPortLabel=else
  Out1 : Outport
  wires:
  In1/1 -> Out1/1
